simulink model "filter_realization"  (R2020b)
settings: Solver=VariableStepAuto  StartTime=0.0  StopTime=20  RelTol=1e-3
settings Model: Creator=153  LastModifiedBy=153

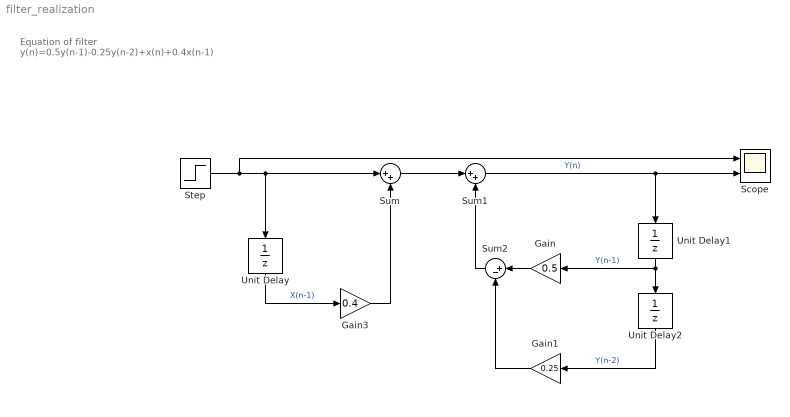
== system filter_realization ==
  note: Equation of filter
      | y(n)=0.5y(n-1)-0.25y(n-2)+x(n)+0.4x(n-1)
  Gain : Gain  Gain=0.5
  Gain1 : Gain  Gain=0.25
  Gain3 : Gain  Gain=0.4
  Scope : Scope  NumInputPorts=2
  Step : Step  SampleTime=0
  Sum : Sum  Inputs=|++
  Sum1 : Sum  Inputs=|++
  Sum2 : Sum  Inputs=|+-
  Unit Delay : UnitDelay  SampleTime=-1  HasFrameUpgradeWarning=on
  Unit Delay1 : UnitDelay  SampleTime=-1  HasFrameUpgradeWarning=on
  Unit Delay2 : UnitDelay  SampleTime=-1  HasFrameUpgradeWarning=on
  wires:
  Gain3/1 -> Sum/2
  Unit Delay/1 -> Gain3/1  "X(n-1)"
  Sum/1 -> Sum1/1
  Sum1/1 -> Unit Delay1/1, Scope/2  "Y(n)"
  Unit Delay1/1 -> Unit Delay2/1, Gain/1  "Y(n-1)"
  Unit Delay2/1 -> Gain1/1  "Y(n-2)"
  Sum2/1 -> Sum1/2
  Gain/1 -> Sum2/1
  Gain1/1 -> Sum2/2
  Step/1 -> Scope/1, Sum/1, Unit Delay/1
